simulink model "Subsystem"  (R2020b)
settings: Solver=VariableStepAuto  StartTime=0.0  StopTime=10.0  RelTol=1e-3
settings Model: Creator=Varun  LastModifiedBy=Varun
settings DataIOCC: SaveOutput=off  SaveTime=off

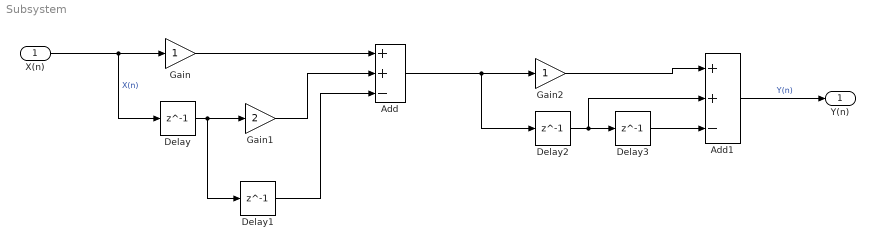
== system Subsystem ==
  X(n) : Inport  OutDataTypeStr=double  PortDimensions=1  SampleTime=[0,1]
  Add : Sum  Inputs=++-
  Add1 : Sum  Inputs=++-
  Delay{,1..3} (4 alike) : Delay  DelayLength=1
  Gain : Gain
  Gain1 : Gain  Gain=2
  Gain2 : Gain
  Y(n) : Outport  OutDataTypeStr=double  PortDimensions=1  SampleTime=[0,1]
  wires:
  Delay3/1 -> Add1/3
  Gain/1 -> Add/1
  Delay1/1 -> Add/3
  X(n)/1 -> Gain/1, Delay/1  "X(n)"
  Gain1/1 -> Add/2
  Add1/1 -> Y(n)/1  "Y(n)"
  Gain2/1 -> Add1/1
  Delay2/1 -> Add1/2, Delay3/1
  Add/1 -> Gain2/1, Delay2/1
  Delay/1 -> Gain1/1, Delay1/1
